simulink model "model_fm2_siso_visual"  (R2025b)
settings: Solver=FixedStepDiscrete  StartTime=0.0  StopTime=100  RelTol=1e-3
undefined symbols (not defined in the file): doppler, magnitude
libraries: commchan3 x2, dspstat3 x2, commdigbbndfm2 x2, commrandsrc3 x1, commsink2 x1
settings Model: Creator=D.mon  LastModifiedBy=D.mon

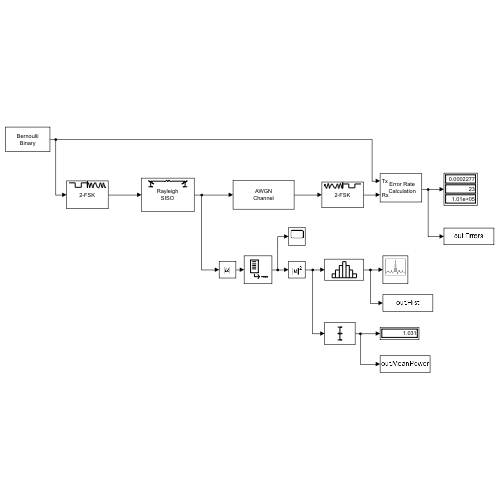
[thumbnail: Simulink's stored preview of the top-level diagram]
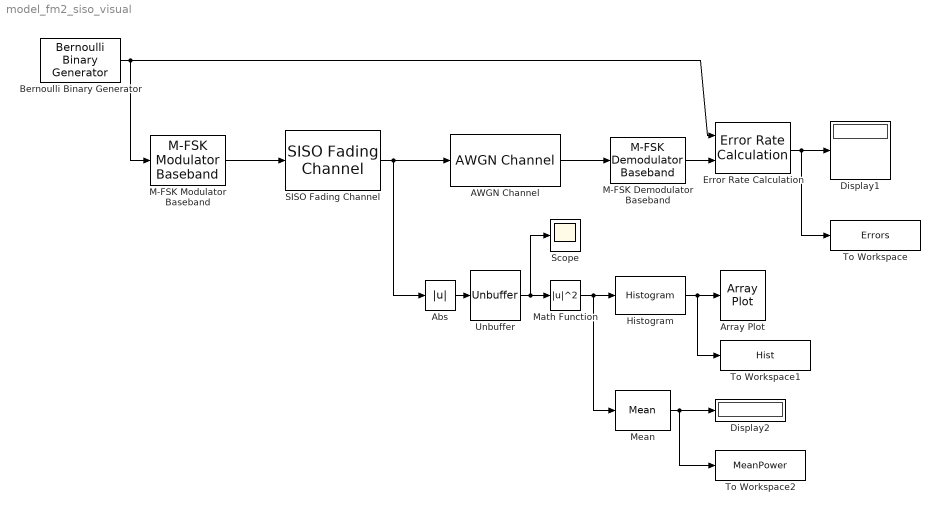
== system model_fm2_siso_visual ==
  AWGN Channel : commchan3/AWGN Channel  LegacyMode=off  NoiseMethod="Signal to noise ratio  (Eb/No)"  noiseMode="Signal to noise ratio  (SNR)"  EbNo=EbPerNo  EsNo=10  SNR=10  BitsPerSymbol=1  SignalPower=1  SpecifySymbolPeriod=off  SamplesPerSymbol=16  SymbolPeriod=1  VarianceSource=Parameter  Variance=1  RandomStream=Global stream  Seed=67  SimulateUsing=Code generation
  Abs : Abs  SaturateOnIntegerOverflow=off
  Array Plot : ArrayPlot  WindowPosition=[959.000000,346.000000,800.000000,500.000000,]  ScopeFrameLocation=window  SampleIncrement=0.1  PlotType=Bar  MaximizeAxes=Off  YLimits=[-0.0151 0.1382]
      settings: OpenAtSimulationStart=off
  Bernoulli Binary Generator : commrandsrc3/Bernoulli Binary Generator  ProbabilityOfZero=0.5  SeedSource=Auto  Seed=0  SampleTime=1e-3  SamplesPerFrame=1000  OutputDataType=double  SimulateUsing=Interpreted execution
  Display1 : Display
  Display2 : Display
  Error Rate Calculation : commsink2/Error Rate Calculation  N=0  st_delay=0  cp_mode=Entire frame  subframe=[]  PMode=Port  WsName=ErrorVec  RsMode2=off  stop=off  numErr=100  maxBits=1e6
  Histogram : dspstat3/Histogram  umin=0  umax=5  nbins=50  operateOver=Each column  Dimension=1  normalized=on  run=on  reset=on  trigtype=None  colComp=on  roundingMode=Floor  overflowMode=off  accumDataTypeStr=Inherit: Same as product output  accumLastDataTypeStr=Inherit: Same as product output
  M-FSK Demodulator Baseband : commdigbbndfm2/M-FSK Demodulator Baseband  M=2  OutType=Integer  Dec=Gray  freqSep=2e3  numSamp=16  RateOptions=Enforce single-rate processing  outDataType=double
  M-FSK Modulator Baseband : commdigbbndfm2/M-FSK Modulator Baseband  M=2  InType=Integer  Enc=Gray  freqSep=2e3  phaseType=Continuous  numSamp=16  RateOptions=Enforce single-rate processing  outDataType=double
  Math Function : Math  Operator=magnitude^2
  Mean : dspstat3/Mean  run=off  InputProcessing=Columns as channels (frame based)  reset_popup=None  directionMode=Each column  dimension=1  roiEnable=off  roiType=Rectangles  roiPortion=Entire ROI  roiOutput=Individual statistics for each ROI  roiFlag=off  roundingMode=Floor  overflowMode=off  outputDataTypeStr=Inherit: Same as accumulator  outputMin=[]  outputMax=[]  outputLastDataTypeStr=Inherit: Same as accumulator
  SISO Fading Channel : commchan3/SISO Fading Channel  InheritSampleRate=on  SampleRate=1  PathDelays=0  AveragePathGains=0  NormalizePathGains=on  FadingDistribution=Rayleigh  KFactor=3  DirectPathDopplerShift=0  DirectPathInitialPhase=0  MaximumDopplerShift=40  DopplerSpectrum=doppler('Jakes')  RandomStream=mt19937ar with seed  Seed=randi(100000)  PathGainsOutputPort=off  ChannelFilterDelayOutputPort=off  SimulateUsing=Interpreted execution  Visualization=Off  PathsForDopplerDisplay=1  SamplesToDisplay=25%
  Scope : Scope
      settings: TimeSpan=0.1  ActiveDisplayYMinimum=0  ActiveDisplayYMaximum=5  DataLoggingMaxPoints=1600  DataLoggingVariableName=Scope
  To Workspace : ToWorkspace  VariableName=Errors  SampleTime=-1
      settings: MaxDataPoints=1
  To Workspace1 : ToWorkspace  VariableName=Hist  SampleTime=-1
      settings: MaxDataPoints=1
  To Workspace2 : ToWorkspace  VariableName=MeanPower  SampleTime=-1
      settings: MaxDataPoints=1
  Unbuffer : Unbuffer
  wires:
  Error Rate Calculation/1 -> To Workspace/1, Display1/1
  Bernoulli Binary Generator/1 -> Error Rate Calculation/1, M-FSK Modulator Baseband/1
  M-FSK Demodulator Baseband/1 -> Error Rate Calculation/2
  M-FSK Modulator Baseband/1 -> SISO Fading Channel/1
  SISO Fading Channel/1 -> Abs/1, AWGN Channel/1
  AWGN Channel/1 -> M-FSK Demodulator Baseband/1
  Abs/1 -> Unbuffer/1
  Unbuffer/1 -> Scope/1, Math Function/1
  Math Function/1 -> Mean/1, Histogram/1
  Histogram/1 -> To Workspace1/1, Array Plot/1
  Mean/1 -> To Workspace2/1, Display2/1
